simulink model "TST_Rail_SetPointAddCor"  (R2016b)
settings: Solver=FixedStepDiscrete  StartTime=0.0  StopTime=simTime  FixedStep=sampleTime  RelTol=1e-3
values from neighbouring files (symbols this model uses):
  testCase = 1    [initTST_Rail_SetPointAddCor_001.m]
libraries: simulink x2
settings Model: Creator=WF305  LastModifiedBy=WF305
settings DebuggingCC: SignalRangeChecking=error

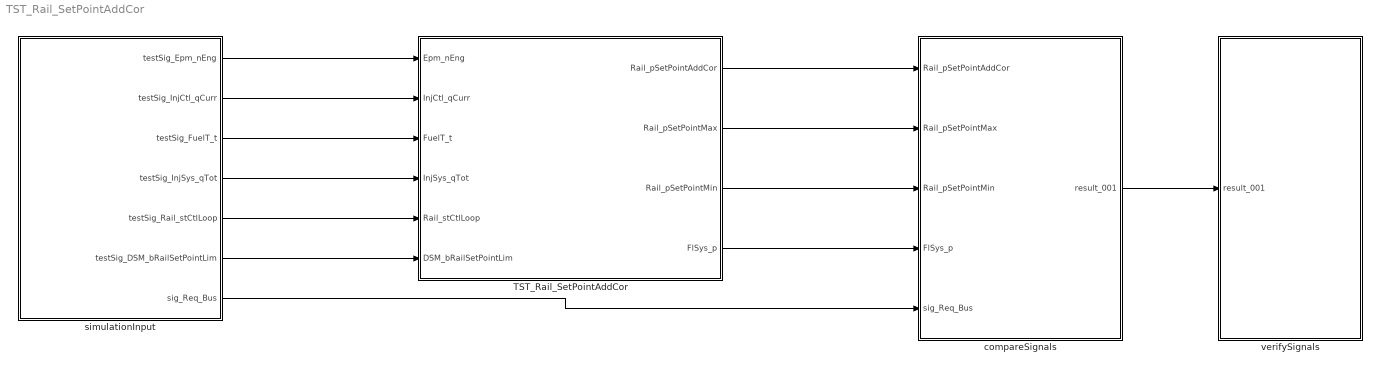
== system TST_Rail_SetPointAddCor ==
  TST_Rail_SetPointAddCor : Subsystem
  compareSignals : Subsystem
  simulationInput : Subsystem
  verifySignals : Subsystem
  wires:
  simulationInput/1(testSig_Epm_nEng) -> TST_Rail_SetPointAddCor/1(Epm_nEng)
  simulationInput/2(testSig_InjCtl_qCurr) -> TST_Rail_SetPointAddCor/2(InjCtl_qCurr)
  simulationInput/3(testSig_FuelT_t) -> TST_Rail_SetPointAddCor/3(FuelT_t)
  simulationInput/4(testSig_InjSys_qTot) -> TST_Rail_SetPointAddCor/4(InjSys_qTot)
  simulationInput/5(testSig_Rail_stCtlLoop) -> TST_Rail_SetPointAddCor/5(Rail_stCtlLoop)
  simulationInput/6(testSig_DSM_bRailSetPointLim) -> TST_Rail_SetPointAddCor/6(DSM_bRailSetPointLim)
  TST_Rail_SetPointAddCor/1(Rail_pSetPointAddCor) -> compareSignals/1(Rail_pSetPointAddCor)
  TST_Rail_SetPointAddCor/2(Rail_pSetPointMax) -> compareSignals/2(Rail_pSetPointMax)
  TST_Rail_SetPointAddCor/3(Rail_pSetPointMin) -> compareSignals/3(Rail_pSetPointMin)
  TST_Rail_SetPointAddCor/4(FlSys_p) -> compareSignals/4(FlSys_p)
  simulationInput/7(sig_Req_Bus) -> compareSignals/5(sig_Req_Bus)
  compareSignals/1(result_001) -> verifySignals/1(result_001)

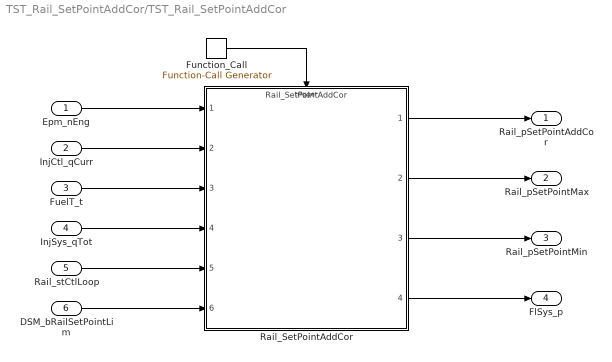
== system TST_Rail_SetPointAddCor/TST_Rail_SetPointAddCor ==
  Epm_nEng : Inport
  InjCtl_qCurr : Inport  Port=2
  FuelT_t : Inport  Port=3
  InjSys_qTot : Inport  Port=4
  Rail_stCtlLoop : Inport  Port=5
  DSM_bRailSetPointLim : Inport  Port=6
  Function_Call : simulink/Ports & Subsystems/Function-Call Generator  sample_time=sampleTime  numberOfIterations=1
  Rail_SetPointAddCor : ModelReference  ModelNameDialog=Rail_SetPointAddCor  ModelReferenceVersion=1.12  TriggerPortName=function  TriggerPortTriggerType=function-call  TriggerPortStatesWhenEnabling=held
  Rail_pSetPointAddCor : Outport
  Rail_pSetPointMax : Outport  Port=2
  Rail_pSetPointMin : Outport  Port=3
  FlSys_p : Outport  Port=4
  wires:
  Function_Call/1 -> Rail_SetPointAddCor/Trigger
  Epm_nEng/1 -> Rail_SetPointAddCor/1
  InjCtl_qCurr/1 -> Rail_SetPointAddCor/2
  FuelT_t/1 -> Rail_SetPointAddCor/3
  InjSys_qTot/1 -> Rail_SetPointAddCor/4
  Rail_stCtlLoop/1 -> Rail_SetPointAddCor/5
  DSM_bRailSetPointLim/1 -> Rail_SetPointAddCor/6
  Rail_SetPointAddCor/1 -> Rail_pSetPointAddCor/1
  Rail_SetPointAddCor/2 -> Rail_pSetPointMax/1
  Rail_SetPointAddCor/3 -> Rail_pSetPointMin/1
  Rail_SetPointAddCor/4 -> FlSys_p/1

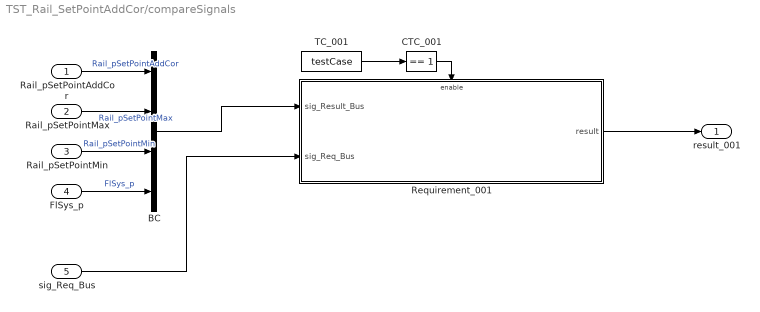
== system TST_Rail_SetPointAddCor/compareSignals ==
  Rail_pSetPointAddCor : Inport
  Rail_pSetPointMax : Inport  Port=2
  Rail_pSetPointMin : Inport  Port=3
  FlSys_p : Inport  Port=4
  sig_Req_Bus : Inport  Port=5
  BC : BusCreator  Inputs=4
  CTC_001 : simulink/Logic and Bit Operations/Compare To Constant  relop===  const=1  OutDataTypeStr=boolean
  Requirement_001 : Subsystem
  TC_001 : Constant  Value=testCase
  result_001 : Outport
  wires:
  Rail_pSetPointAddCor/1 -> BC/1  "Rail_pSetPointAddCor"
  Rail_pSetPointMax/1 -> BC/2  "Rail_pSetPointMax"
  Rail_pSetPointMin/1 -> BC/3  "Rail_pSetPointMin"
  FlSys_p/1 -> BC/4  "FlSys_p"
  TC_001/1 -> CTC_001/1
  CTC_001/1 -> Requirement_001/Enable
  sig_Req_Bus/1 -> Requirement_001/2(sig_Req_Bus)
  BC/1 -> Requirement_001/1(sig_Result_Bus)
  Requirement_001/1(result) -> result_001/1

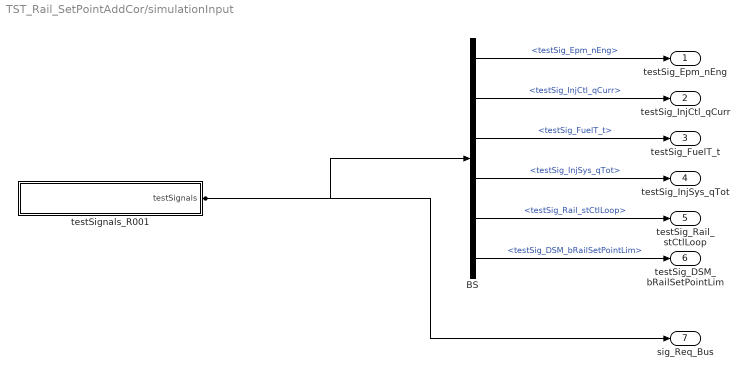
== system TST_Rail_SetPointAddCor/simulationInput ==
  BS : BusSelector  OutputSignals=testSig_Epm_nEng,testSig_InjCtl_qCurr,testSig_FuelT_t,testSig_InjSys_qTot,testSig_Rail_stCtlLoop,testSig_DSM_bRailSetPointLim
  testSignals_R001 : Subsystem
  testSig_Epm_nEng : Outport
  testSig_InjCtl_qCurr : Outport  Port=2
  testSig_FuelT_t : Outport  Port=3
  testSig_InjSys_qTot : Outport  Port=4
  testSig_Rail_stCtlLoop : Outport  Port=5
  testSig_DSM_bRailSetPointLim : Outport  Port=6
  sig_Req_Bus : Outport  Port=7
  wires:
  BS/1 -> testSig_Epm_nEng/1  "<testSig_Epm_nEng>"
  BS/2 -> testSig_InjCtl_qCurr/1  "<testSig_InjCtl_qCurr>"
  BS/3 -> testSig_FuelT_t/1  "<testSig_FuelT_t>"
  BS/4 -> testSig_InjSys_qTot/1  "<testSig_InjSys_qTot>"
  BS/5 -> testSig_Rail_stCtlLoop/1  "<testSig_Rail_stCtlLoop>"
  BS/6 -> testSig_DSM_bRailSetPointLim/1  "<testSig_DSM_bRailSetPointLim>"
  testSignals_R001/1(testSignals) -> BS/1, sig_Req_Bus/1

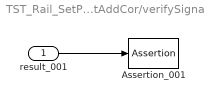
== system TST_Rail_SetPointAddCor/verifySignals ==
  result_001 : Inport
  Assertion_001 : Assertion  Enabled=off
  wires:
  result_001/1 -> Assertion_001/1

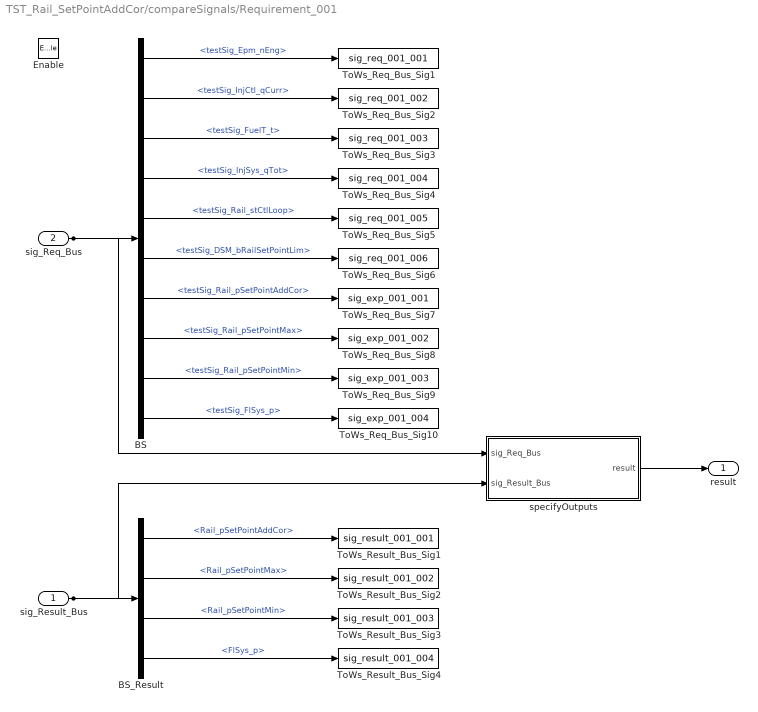
== system TST_Rail_SetPointAddCor/compareSignals/Requirement_001 ==
  sig_Result_Bus : Inport
  sig_Req_Bus : Inport  Port=2
  Enable : EnablePort
  BS : BusSelector  OutputSignals=testSig_Epm_nEng,testSig_InjCtl_qCurr,testSig_FuelT_t,testSig_InjSys_qTot,testSig_Rail_stCtlLoop,testSig_DSM_bRailSetPointLim,testSig_Rail_pSetPointAddCor,testSig_Rail_pSetPointMax,testSig_Rail_pSetPointMin,testSig_FlSys_p
  BS_Result : BusSelector  OutputSignals=Rail_pSetPointAddCor,Rail_pSetPointMax,Rail_pSetPointMin,FlSys_p
  ToWs_Req_Bus_Sig1 : ToWorkspace  VariableName=sig_req_001_001  SaveFormat=Structure With Time
  ToWs_Req_Bus_Sig10 : ToWorkspace  VariableName=sig_exp_001_004  SaveFormat=Structure With Time
  ToWs_Req_Bus_Sig2 : ToWorkspace  VariableName=sig_req_001_002  SaveFormat=Structure With Time
  ToWs_Req_Bus_Sig3 : ToWorkspace  VariableName=sig_req_001_003  SaveFormat=Structure With Time
  ToWs_Req_Bus_Sig4 : ToWorkspace  VariableName=sig_req_001_004  SaveFormat=Structure With Time
  ToWs_Req_Bus_Sig5 : ToWorkspace  VariableName=sig_req_001_005  SaveFormat=Structure With Time
  ToWs_Req_Bus_Sig6 : ToWorkspace  VariableName=sig_req_001_006  SaveFormat=Structure With Time
  ToWs_Req_Bus_Sig7 : ToWorkspace  VariableName=sig_exp_001_001  SaveFormat=Structure With Time
  ToWs_Req_Bus_Sig8 : ToWorkspace  VariableName=sig_exp_001_002  SaveFormat=Structure With Time
  ToWs_Req_Bus_Sig9 : ToWorkspace  VariableName=sig_exp_001_003  SaveFormat=Structure With Time
  ToWs_Result_Bus_Sig1 : ToWorkspace  VariableName=sig_result_001_001  SaveFormat=Structure With Time
  ToWs_Result_Bus_Sig2 : ToWorkspace  VariableName=sig_result_001_002  SaveFormat=Structure With Time
  ToWs_Result_Bus_Sig3 : ToWorkspace  VariableName=sig_result_001_003  SaveFormat=Structure With Time
  ToWs_Result_Bus_Sig4 : ToWorkspace  VariableName=sig_result_001_004  SaveFormat=Structure With Time
  specifyOutputs : Subsystem
  result : Outport
  wires:
  sig_Req_Bus/1 -> BS/1, specifyOutputs/1(sig_Req_Bus)
  BS/1 -> ToWs_Req_Bus_Sig1/1  "<testSig_Epm_nEng>"
  BS/2 -> ToWs_Req_Bus_Sig2/1  "<testSig_InjCtl_qCurr>"
  BS/3 -> ToWs_Req_Bus_Sig3/1  "<testSig_FuelT_t>"
  BS/4 -> ToWs_Req_Bus_Sig4/1  "<testSig_InjSys_qTot>"
  BS/5 -> ToWs_Req_Bus_Sig5/1  "<testSig_Rail_stCtlLoop>"
  BS/6 -> ToWs_Req_Bus_Sig6/1  "<testSig_DSM_bRailSetPointLim>"
  BS/7 -> ToWs_Req_Bus_Sig7/1  "<testSig_Rail_pSetPointAddCor>"
  BS/8 -> ToWs_Req_Bus_Sig8/1  "<testSig_Rail_pSetPointMax>"
  BS/9 -> ToWs_Req_Bus_Sig9/1  "<testSig_Rail_pSetPointMin>"
  BS/10 -> ToWs_Req_Bus_Sig10/1  "<testSig_FlSys_p>"
  sig_Result_Bus/1 -> BS_Result/1, specifyOutputs/2(sig_Result_Bus)
  BS_Result/1 -> ToWs_Result_Bus_Sig1/1  "<Rail_pSetPointAddCor>"
  BS_Result/2 -> ToWs_Result_Bus_Sig2/1  "<Rail_pSetPointMax>"
  BS_Result/3 -> ToWs_Result_Bus_Sig3/1  "<Rail_pSetPointMin>"
  BS_Result/4 -> ToWs_Result_Bus_Sig4/1  "<FlSys_p>"
  specifyOutputs/1(result) -> result/1

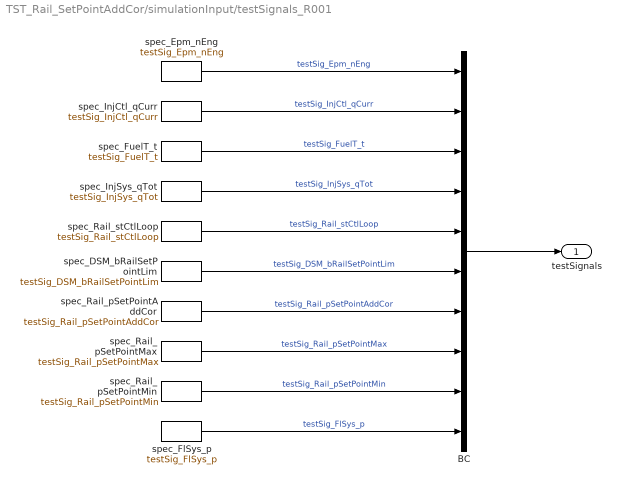
== system TST_Rail_SetPointAddCor/simulationInput/testSignals_R001 ==
  BC : BusCreator  Inputs=10
  spec_DSM_bRailSetPointLim : FromWorkspace  VariableName=testSig_DSM_bRailSetPointLim  Interpolate=off  OutputAfterFinalValue=Holding final value
  spec_Epm_nEng : FromWorkspace  VariableName=testSig_Epm_nEng  Interpolate=off  OutputAfterFinalValue=Holding final value
  spec_FlSys_p : FromWorkspace  VariableName=testSig_FlSys_p  Interpolate=off  OutputAfterFinalValue=Holding final value
  spec_FuelT_t : FromWorkspace  VariableName=testSig_FuelT_t  Interpolate=off  OutputAfterFinalValue=Holding final value
  spec_InjCtl_qCurr : FromWorkspace  VariableName=testSig_InjCtl_qCurr  Interpolate=off  OutputAfterFinalValue=Holding final value
  spec_InjSys_qTot : FromWorkspace  VariableName=testSig_InjSys_qTot  Interpolate=off  OutputAfterFinalValue=Holding final value
  spec_Rail_pSetPointAddCor : FromWorkspace  VariableName=testSig_Rail_pSetPointAddCor  Interpolate=off  OutputAfterFinalValue=Holding final value
  spec_Rail_pSetPointMax : FromWorkspace  VariableName=testSig_Rail_pSetPointMax  Interpolate=off  OutputAfterFinalValue=Holding final value
  spec_Rail_pSetPointMin : FromWorkspace  VariableName=testSig_Rail_pSetPointMin  Interpolate=off  OutputAfterFinalValue=Holding final value
  spec_Rail_stCtlLoop : FromWorkspace  VariableName=testSig_Rail_stCtlLoop  Interpolate=off  OutputAfterFinalValue=Holding final value
  testSignals : Outport
  wires:
  BC/1 -> testSignals/1
  spec_Epm_nEng/1 -> BC/1  "testSig_Epm_nEng"
  spec_InjCtl_qCurr/1 -> BC/2  "testSig_InjCtl_qCurr"
  spec_FuelT_t/1 -> BC/3  "testSig_FuelT_t"
  spec_InjSys_qTot/1 -> BC/4  "testSig_InjSys_qTot"
  spec_Rail_stCtlLoop/1 -> BC/5  "testSig_Rail_stCtlLoop"
  spec_DSM_bRailSetPointLim/1 -> BC/6  "testSig_DSM_bRailSetPointLim"
  spec_Rail_pSetPointAddCor/1 -> BC/7  "testSig_Rail_pSetPointAddCor"
  spec_Rail_pSetPointMax/1 -> BC/8  "testSig_Rail_pSetPointMax"
  spec_Rail_pSetPointMin/1 -> BC/9  "testSig_Rail_pSetPointMin"
  spec_FlSys_p/1 -> BC/10  "testSig_FlSys_p"

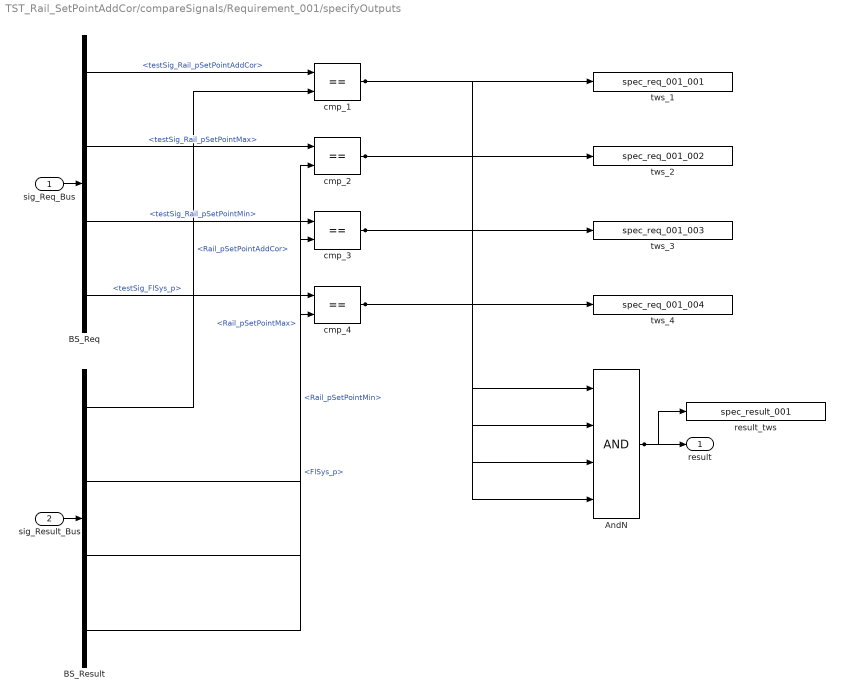
== system TST_Rail_SetPointAddCor/compareSignals/Requirement_001/specifyOutputs ==
  sig_Req_Bus : Inport
  sig_Result_Bus : Inport  Port=2
  AndN : Logic  Inputs=4
  BS_Req : BusSelector  OutputSignals=testSig_Rail_pSetPointAddCor,testSig_Rail_pSetPointMax,testSig_Rail_pSetPointMin,testSig_FlSys_p
  BS_Result : BusSelector  OutputSignals=Rail_pSetPointAddCor,Rail_pSetPointMax,Rail_pSetPointMin,FlSys_p
  cmp_{1..4} (4 alike) : RelationalOperator  Operator===  RndMeth=Nearest  InputSameDT=on
  result_tws : ToWorkspace  VariableName=spec_result_001
  tws_1 : ToWorkspace  VariableName=spec_req_001_001
  tws_2 : ToWorkspace  VariableName=spec_req_001_002
  tws_3 : ToWorkspace  VariableName=spec_req_001_003
  tws_4 : ToWorkspace  VariableName=spec_req_001_004
  result : Outport
  wires:
  sig_Req_Bus/1 -> BS_Req/1
  sig_Result_Bus/1 -> BS_Result/1
  AndN/1 -> result/1, result_tws/1
  BS_Req/1 -> cmp_1/1  "<testSig_Rail_pSetPointAddCor>"
  BS_Result/1 -> cmp_1/2  "<Rail_pSetPointAddCor>"
  cmp_1/1 -> tws_1/1, AndN/1
  BS_Req/2 -> cmp_2/1  "<testSig_Rail_pSetPointMax>"
  BS_Result/2 -> cmp_2/2  "<Rail_pSetPointMax>"
  cmp_2/1 -> tws_2/1, AndN/2
  BS_Req/3 -> cmp_3/1  "<testSig_Rail_pSetPointMin>"
  BS_Result/3 -> cmp_3/2  "<Rail_pSetPointMin>"
  cmp_3/1 -> tws_3/1, AndN/3
  BS_Req/4 -> cmp_4/1  "<testSig_FlSys_p>"
  BS_Result/4 -> cmp_4/2  "<FlSys_p>"
  cmp_4/1 -> tws_4/1, AndN/4
